simulink model "no-pid"  (R2022a)
settings: Solver=FixedStepAuto  StartTime=0.0  StopTime=10  RelTol=1e-3
settings Model: Creator=yfx13  LastModifiedBy=yfx13

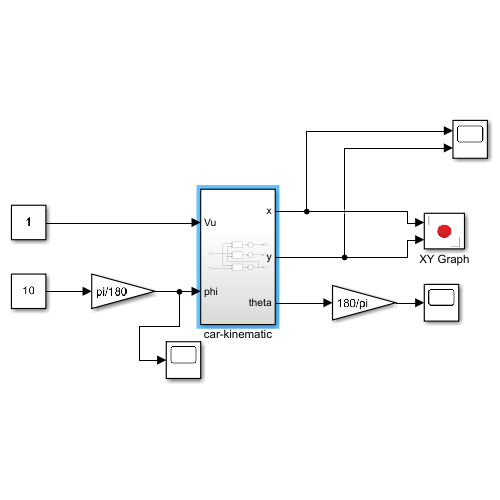
[thumbnail: Simulink's stored preview of the top-level diagram]
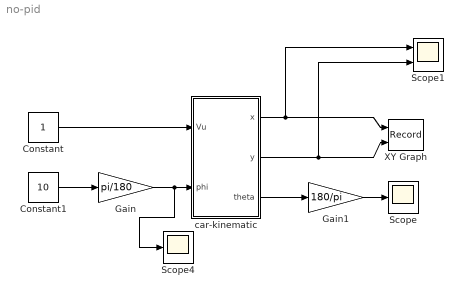
== system no-pid ==
  Constant : Constant
  Constant1 : Constant  Value=10
  Gain : Gain  Gain=pi/180
  Gain1 : Gain  Gain=180/pi
  Scope : Scope
  Scope1 : Scope  NumInputPorts=2
  Scope4 : Scope
  XY Graph : Record  FileSettingsInternal="{\"entries\":[{\"content\":{\"excelSettings\":{\"content\":{},\"type\":\"Streamout.ExcelSettings\"}},\"type\":\"Streamout.FileSettingStorage\",\"uuid\":\"09be61e3-095a-4077-83e3-235673339609\"}],\"packageUris\":[\"http://schema.mathworks.com/mf0/streamout_blocks/R2020a\"],\"version\":\"1.0\"}"  Layout=[1 1]  SignalsInternal="{\"entries\":[{\"content\":{\"signals\":[{\"content\":{\"blockPath\":[\"test/XY Graph\"],\"channel\":[],\"dimensions\":[1],\"domain\":\"test/XY Graph\",\"lineColor\":\"#a2142f\",\"plots\":[1],\"port\":1,\"sid\":[\"\"],\"signalID\":20,\"signalName\":\"car-kinematic:1\"},\"type\":\"RecordBlkView.Signal\",\"uuid\":\"8ade2e4c-d0c5-4669-8e9e-364c20c690cf\"},{\"content\":{\"blockPath\":[\"test/XY Graph\"],\"channel\":[],\"dimensions\":[1],\"domain\":\"test/XY Graph\",\"lineColor\":\"#139fff\",\"plots\":[1],\"port\":2,\"sid\":[\"\"],\"signalID\":24,\"signalName\":\"car-kinematic:2\"},\"type\":\"RecordBlkView.Signal\",\"uuid\":\"59ec11ac-7cb7-480e-908e-b4479f66b96c\"}]},\"type\":\"RecordBlkView.InputSignals\",\"uuid\":\"938a61be-d039-471a-8541-1b2cbd6061d6\"}],\"packageUris\":[\"http://schema.mathworks.com/mf0/streamout_blocks/R2020a\"],\"version\":\"1.0\"}"  VisualizationBindings="{\"xyplotplugin\":{\"info\":[{\"series\":[{\"bindingParametersList\":[{\"parameter\":\"X-Axis\",\"signalID\":20,\"signalName\":\"car-kinematic:1\"},{\"parameter\":\"Y-Axis\",\"signalID\":24,\"signalName\":\"car-kinematic:2\"}],\"seriesID\":16430}],\"subplotID\":1}]}}"  CompatibilityTag=XY
  car-kinematic : Subsystem
  wires:
  Gain1/1 -> Scope/1
  Constant/1 -> car-kinematic/1(Vu)
  car-kinematic/3(theta) -> Gain1/1
  car-kinematic/1(x) -> XY Graph/1, Scope1/1
  car-kinematic/2(y) -> Scope1/2, XY Graph/2
  Constant1/1 -> Gain/1
  Gain/1 -> Scope4/1, car-kinematic/2(phi)

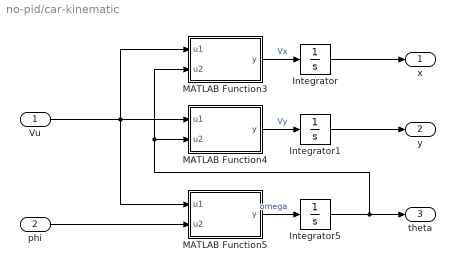
== system no-pid/car-kinematic ==
  Vu : Inport
  phi : Inport  Port=2
  Integrator : Integrator
  Integrator1 : Integrator
  Integrator5 : Integrator
  MATLAB Function3 : MATLAB Function  TreatAsAtomicUnit=on
  MATLAB Function4 : MATLAB Function  TreatAsAtomicUnit=on
  MATLAB Function5 : MATLAB Function  TreatAsAtomicUnit=on
  x : Outport
  y : Outport  Port=2
  theta : Outport  Port=3
  wires:
  Integrator5/1 -> MATLAB Function4/2(u2), MATLAB Function3/2(u2), theta/1
  MATLAB Function5/1(y) -> Integrator5/1  "omega"
  Vu/1 -> MATLAB Function5/1(u1), MATLAB Function4/1(u1), MATLAB Function3/1(u1)
  phi/1 -> MATLAB Function5/2(u2)
  MATLAB Function3/1(y) -> Integrator/1  "Vx"
  Integrator/1 -> x/1
  MATLAB Function4/1(y) -> Integrator1/1  "Vy"
  Integrator1/1 -> y/1

== matlab function no-pid/car-kinematic/MATLAB Function4 ==
  data: u1 input; y output; u2 input
function y = fcn(u1,u2)
y=u1*sin(u2);

== matlab function no-pid/car-kinematic/MATLAB Function5 ==
  data: u1 input; y output; u2 input
function y = fcn(u1,u2)
L=10*2.54/100;
y=u1*tan(u2)/L;

== matlab function no-pid/car-kinematic/MATLAB Function3 ==
  data: u1 input; y output; u2 input
function y = fcn(u1,u2)
y=u1*cos(u2);
